simulink model "t27"  (R2024b)
settings: Solver=ode45  StartTime=0.0  StopTime=20.0  RelTol=1e-3
settings Model: Creator=lenovo  LastModifiedBy=lenovo

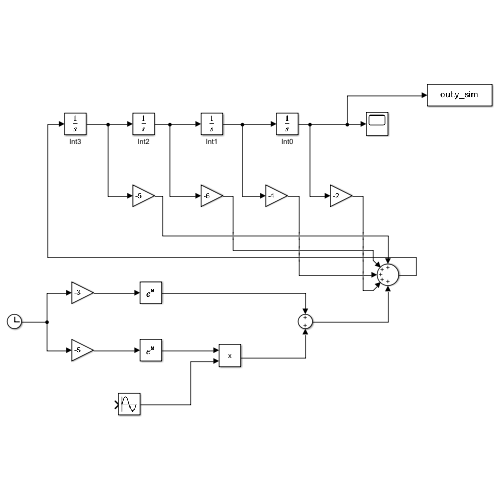
[thumbnail: Simulink's stored preview of the top-level diagram]
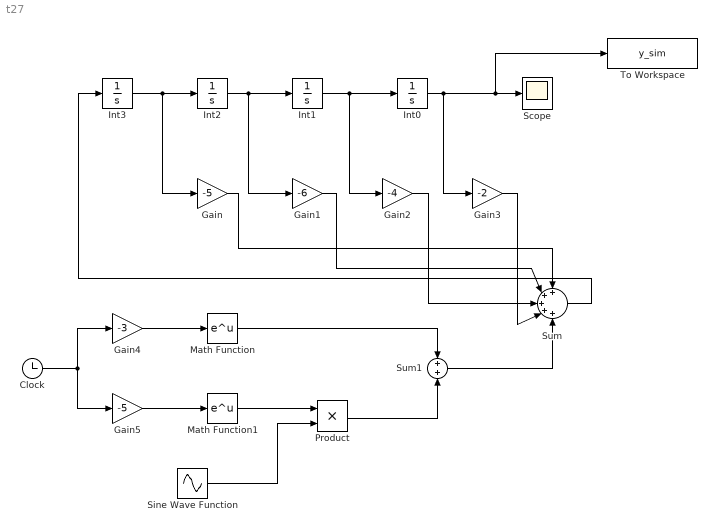
== system t27 ==
  Clock : Clock
  Gain : Gain  Gain=-5
  Gain1 : Gain  Gain=-6
  Gain2 : Gain  Gain=-4
  Gain3 : Gain  Gain=-2
  Gain4 : Gain  Gain=-3
  Gain5 : Gain  Gain=-5
  Int0 : Integrator  InitialCondition=1  ContinuousStateAttributes='Int0'
  Int1 : Integrator  InitialCondition=0.5  ContinuousStateAttributes='Int1'
  Int2 : Integrator  InitialCondition=0.5  ContinuousStateAttributes='Int2'
  Int3 : Integrator  InitialCondition=0.2  ContinuousStateAttributes='Int3'
  Math Function : Math
  Math Function1 : Math
  Product : Product
  Scope : Scope
  Sine Wave Function : Sin  TimeSource=Use external signal  Frequency=4  Phase=pi/3  SampleTime=0
  Sum : Sum  Inputs=+++++
  Sum1 : Sum
  To Workspace : ToWorkspace  VariableName=y_sim  SaveFormat=Structure With Time  SampleTime=-1
  wires:
  Int3/1 -> Gain/1, Int2/1
  Int2/1 -> Gain1/1, Int1/1
  Int1/1 -> Gain2/1, Int0/1
  Int0/1 -> To Workspace/1, Scope/1, Gain3/1
  Gain/1 -> Sum/1
  Gain1/1 -> Sum/2
  Gain2/1 -> Sum/3
  Gain3/1 -> Sum/4
  Clock/1 -> Gain5/1, Gain4/1
  Gain4/1 -> Math Function/1
  Gain5/1 -> Math Function1/1
  Math Function1/1 -> Product/1
  Sine Wave Function/1 -> Product/2
  Math Function/1 -> Sum1/1
  Product/1 -> Sum1/2
  Sum1/1 -> Sum/5
  Sum/1 -> Int3/1
